simulink model "airspeed_hold_using_commanded_throttle"  (Simulink 7.7)
settings: Solver=ode45  StartTime=0.0  StopTime=10.0  RelTol=1e-3
undefined symbols (not defined in the file): a_V_1, a_V_2, k_i_V, k_p_V
settings Model: Creator=prattmic  LastModifiedBy=prattmic

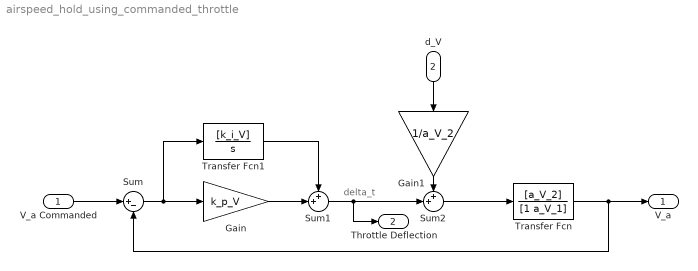
== system airspeed_hold_using_commanded_throttle ==
  note: delta_t
  V_a Commanded : Inport
  d_V : Inport  Port=2
  Gain : Gain  Gain=k_p_V
  Gain1 : Gain  Gain=1/a_V_2
  Sum : Sum  Inputs=|+-
  Sum1 : Sum  Inputs=++|
  Sum2 : Sum  Inputs=++|
  Transfer Fcn : TransferFcn  Numerator=[a_V_2]  Denominator=[1 a_V_1]
  Transfer Fcn1 : TransferFcn  Numerator=[k_i_V]  Denominator=[1 0]
  V_a : Outport
  Throttle Deflection : Outport  Port=2
  wires:
  d_V/1 -> Gain1/1
  Gain1/1 -> Sum2/1
  Transfer Fcn1/1 -> Sum1/1
  V_a Commanded/1 -> Sum/1
  Sum/1 -> Gain/1, Transfer Fcn1/1
  Gain/1 -> Sum1/2
  Sum1/1 -> Sum2/2, Throttle Deflection/1
  Sum2/1 -> Transfer Fcn/1
  Transfer Fcn/1 -> V_a/1, Sum/2
